simulink model "sevensegmentdisplay"  (R2024a)
settings: Solver=VariableStepAuto  StartTime=0.0  StopTime=10.0  RelTol=1e-3
settings Model: Creator=prath  LastModifiedBy=prath

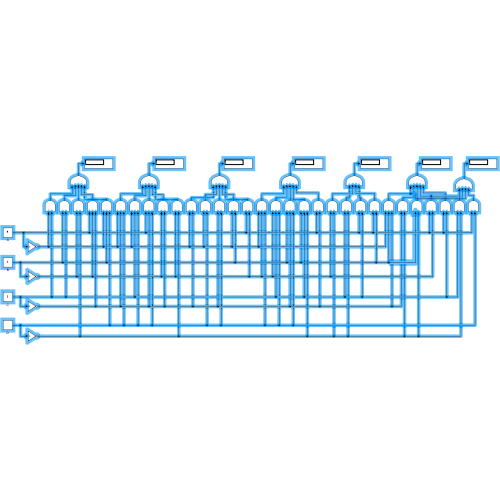
[thumbnail: Simulink's stored preview of the top-level diagram]
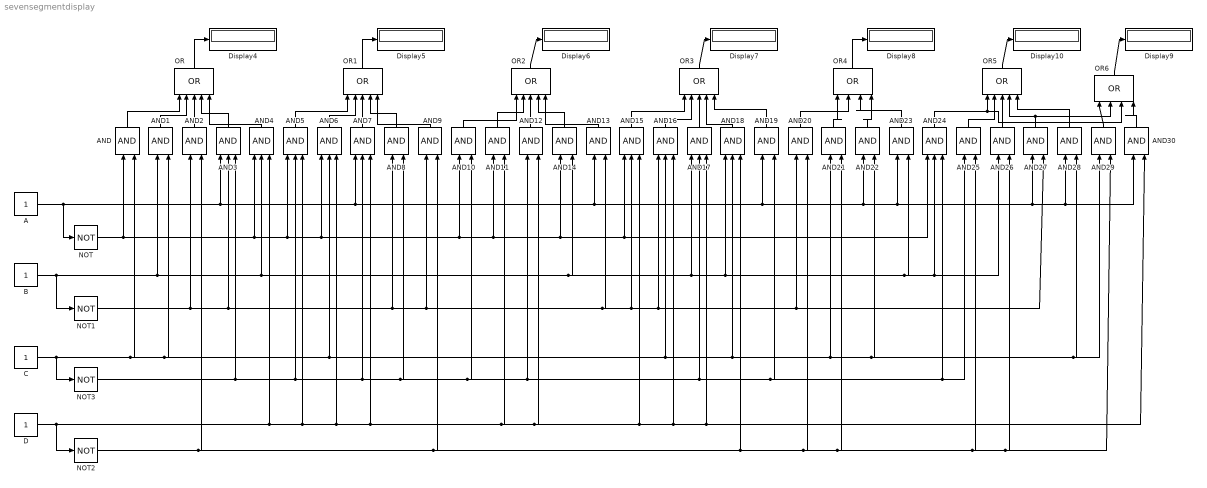
== system sevensegmentdisplay ==
  A : Constant
  AND{,1..2,8..14,19..23,25..30} (21 alike) : Logic  IconShape=distinctive  AllPortsSameDT=off  OutDataTypeStr=boolean
  AND{3..7,15..18,24} (10 alike) : Logic  Inputs=3  IconShape=distinctive  AllPortsSameDT=off  OutDataTypeStr=boolean
  B : Constant
  C : Constant
  D : Constant
  Display{4..10} (7 alike) : Display
  NOT{,1..3} (4 alike) : Logic  Operator=NOT  IconShape=distinctive  AllPortsSameDT=off  OutDataTypeStr=boolean
  OR{,1..3,5} (5 alike) : Logic  Operator=OR  Inputs=5  IconShape=distinctive  AllPortsSameDT=off  OutDataTypeStr=boolean
  OR4 : Logic  Operator=OR  Inputs=4  IconShape=distinctive  AllPortsSameDT=off  OutDataTypeStr=boolean
  OR6 : Logic  Operator=OR  Inputs=4  IconShape=distinctive  AllPortsSameDT=off  OutDataTypeStr=boolean
  wires:
  AND30/1 -> OR6/4
  AND7/1 -> OR1/3
  OR3/1 -> Display7/1
  AND2/1 -> OR/3
  AND6/1 -> OR1/2
  AND25/1 -> OR5/2
  AND17/1 -> OR3/3
  AND28/1 -> OR5/5
  AND19/1 -> OR3/5
  OR2/1 -> Display6/1
  AND13/1 -> OR2/5
  OR/1 -> Display4/1
  AND3/1 -> OR/4
  OR1/1 -> Display5/1
  AND20/1 -> OR4/2
  OR5/1 -> Display10/1
  NOT2/1 -> AND29/2, AND26/2, AND25/2, AND21/2, AND20/2, AND18/3, AND9/2, AND2/2
  AND12/1 -> OR2/3
  OR4/1 -> Display8/1
  AND27/1 -> OR5/4, OR6/2
  AND11/1 -> OR2/2
  AND14/1 -> OR2/4
  AND5/1 -> OR1/1
  AND16/1 -> OR3/2
  AND21/1 -> OR4/1
  NOT3/1 -> AND25/1, AND24/3, AND19/2, AND17/2, AND12/1, AND10/2, AND8/2, AND7/2, AND5/2, AND3/3
  AND/1 -> OR/1
  AND8/1 -> OR1/4
  AND24/1 -> OR6/3, OR5/1
  AND10/1 -> OR2/1
  C/1 -> AND29/1, AND28/2, AND22/2, AND21/1, AND18/2, AND16/2, AND6/2, AND1/2, AND/2, NOT3/1
  OR6/1 -> Display9/1
  AND29/1 -> OR6/1
  A/1 -> AND30/1, AND28/1, AND27/1, AND23/1, AND22/1, AND19/1, AND13/1, AND7/1, AND3/1, NOT/1
  AND15/1 -> OR3/1
  AND4/1 -> OR/5
  NOT1/1 -> AND27/2, AND20/1, AND16/1, AND15/2, AND13/2, AND9/1, AND8/1, AND3/2, AND2/1
  AND18/1 -> OR3/4
  AND9/1 -> OR1/5
  AND1/1 -> OR/2
  AND23/1 -> OR4/3
  AND22/1 -> OR4/4
  NOT/1 -> AND24/1, AND15/1, AND14/1, AND11/1, AND10/1, AND6/1, AND5/1, AND4/1, AND/1
  AND26/1 -> OR5/3
  D/1 -> AND30/2, AND17/3, AND16/3, AND15/3, AND12/2, AND11/2, AND7/3, AND6/3, AND5/3, AND4/3, NOT2/1
  B/1 -> AND26/1, AND24/2, AND23/2, AND18/1, AND17/1, AND14/2, AND4/2, AND1/1, NOT1/1
